simulink model "control_mixing_s"  (R2014b)
settings: Solver=ode45  SolverMode=SingleTasking  StartTime=0.0  StopTime=10.0  RelTol=1e-3
settings Model: TunableVars=quadModel  TunableVarsStorageClass=Auto  Creator=magogs00  LastModifiedBy=magogs00
settings DataIOCC: SaveFormat=Structure  SaveOutput=off  SaveTime=off
settings OptimizationCC: BlockReduction=off  BooleanDataType=off  InlineParams=on
settings DebuggingCC: UnderspecifiedInitializationDetection=Classic  MergeDetectMultiDrivingBlocksExec=none  SignalResolutionControl=TryResolveAll

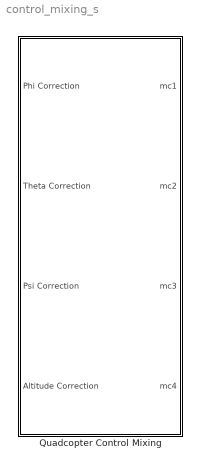
== system control_mixing_s ==
  Quadcopter Control Mixing : Subsystem
      mask help: Simulink:masks:GenSFuncDesc_MD
      mask Help: eval('feval(''rtwprivate'',''rtwhelpview'',''rtw_sfcn_block'')');
      mask Display:
      | modelLoaded = evalin('base','exist(''quadModel'',''var'')');
      | if (modelLoaded==1)
      |     if (evalin('base','quadModel.plusConfig'))
      |     fprintf([' \n' ' \n'  'Configuration "+"']);
      |     else if (~evalin('base','quadModel.plusConfig'))
      |         fprintf([' \n' ' \n' 'Configuration "X"']);
      |         end
      |     end
      | else
      |     fprintf([' \n' ' \n'  'Model Not Loaded']);
      | end

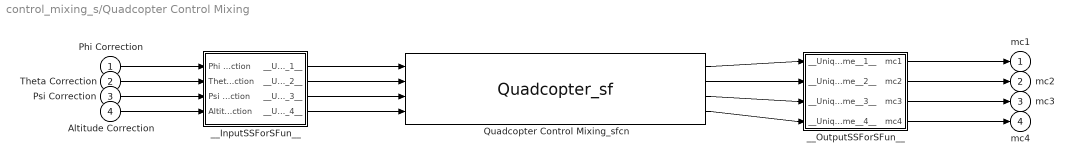
== system control_mixing_s/Quadcopter Control Mixing ==
  Phi Correction : Inport
  Theta Correction : Inport  Port=2
  Psi Correction : Inport  Port=3
  Altitude Correction : Inport  Port=4
  Quadcopter Control Mixing_sfcn : S-Function  FunctionName=Quadcopter_sf  SFunctionModules=""  EnableBusSupport=off  mask{rtw_sf_name=Quadcopter_sf, showVar=off}
      mask prompts: rtw_sf_name "Simulink:masks:GenSFuncName_MP"; showVar "Simulink:masks:GenSFuncShowModuleList_MP"
      mask help: Simulink:masks:GenSFuncDesc_MD
      mask init:
      | displist = '';
      | if ~strcmp(get_param(gcb, 'FunctionName'), rtw_sf_name);
      |   set_param(gcb, 'FunctionName', rtw_sf_name);
      | end
      | % Check if we are generating code
      | rtw_mode = false;
      | if strcmpi(get_param(bdroot(gcb),'SimulationStatus'),'Initializing')
      | 	rtw_mode = strcmpi(get_param(bdroot(gcb),'BuildingRTWCode'),'on') && ...
      | 		~strcmpi(get_param(bdroot(gcb),'TargetStyle'),'SimulationTarget');
      | end
      | if showVar || rtw_mode
      | 	if exist('rtwsfunc') == 2 | exist('rtwsfunc') == 6
      | 		tmplist = rtwsfunc(rtw_sf_name,gcb);
      | 		tmplist = DAStudio.message('Simulink:masks:GenSFuncListOfModules_IC', tmplist);
      | 	elseif showVar
      | 		tmplist1 = DAStudio.message('Simulink:masks:GenSFuncListOfModules_IC', '');
      |         tmplist2 = DAStudio.message('Simulink:masks:GenSFuncNotLicensed_IC');
      |         tmplist = [tmplist1 tmplist2];
      |  	end
      | end
      | if showVar
      |   displist = tmplist;
      | end
      settings: CopyFcn=|
      | if ~strcmp(get_param(gcb,'Linkstatus'),'none') && ...
      | ~strcmp(get_param(gcb,'Linkstatus'),'implicit')
      |   set_param(gcb,'LinkStatus','none');
      | end
      mask Help: eval('feval(''rtwprivate'',''rtwhelpview'',''rtw_sfcn_block'')');
      mask Display:
      | port_label('input',1,'Phi Correction');
      | port_label('input',2,'Theta Correction');
      | port_label('input',3,'Psi Correction');
      | port_label('input',4,'Altitude Correction');
      | port_label('output',1,'mc1');
      | port_label('output',2,'mc2');
      | port_label('output',3,'mc3');
      | port_label('output',4,'mc4');
  __InputSSForSFun__ : Subsystem
  __OutputSSForSFun__ : Subsystem
  mc1 : Outport
  mc2 : Outport  Port=2
  mc3 : Outport  Port=3
  mc4 : Outport  Port=4
  wires:
  Phi Correction/1 -> __InputSSForSFun__/1(Phi Correction)
  Theta Correction/1 -> __InputSSForSFun__/2(Theta Correction)
  Psi Correction/1 -> __InputSSForSFun__/3(Psi Correction)
  Altitude Correction/1 -> __InputSSForSFun__/4(Altitude Correction)
  __InputSSForSFun__/1(__UniqueOutportName__1__) -> Quadcopter Control Mixing_sfcn/1
  __InputSSForSFun__/2(__UniqueOutportName__2__) -> Quadcopter Control Mixing_sfcn/2
  __InputSSForSFun__/3(__UniqueOutportName__3__) -> Quadcopter Control Mixing_sfcn/3
  __InputSSForSFun__/4(__UniqueOutportName__4__) -> Quadcopter Control Mixing_sfcn/4
  Quadcopter Control Mixing_sfcn/1 -> __OutputSSForSFun__/1(__UniqueInportName__1__)
  Quadcopter Control Mixing_sfcn/2 -> __OutputSSForSFun__/2(__UniqueInportName__2__)
  Quadcopter Control Mixing_sfcn/3 -> __OutputSSForSFun__/3(__UniqueInportName__3__)
  Quadcopter Control Mixing_sfcn/4 -> __OutputSSForSFun__/4(__UniqueInportName__4__)
  __OutputSSForSFun__/1(mc1) -> mc1/1
  __OutputSSForSFun__/2(mc2) -> mc2/1
  __OutputSSForSFun__/3(mc3) -> mc3/1
  __OutputSSForSFun__/4(mc4) -> mc4/1

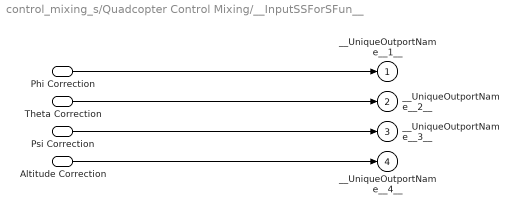
== system control_mixing_s/Quadcopter Control Mixing/__InputSSForSFun__ ==
  Phi Correction : Inport
  Theta Correction : Inport  Port=2
  Psi Correction : Inport  Port=3
  Altitude Correction : Inport  Port=4
  __UniqueOutportName__1__ : Outport
  __UniqueOutportName__2__ : Outport  Port=2
  __UniqueOutportName__3__ : Outport  Port=3
  __UniqueOutportName__4__ : Outport  Port=4
  wires:
  Phi Correction/1 -> __UniqueOutportName__1__/1
  Theta Correction/1 -> __UniqueOutportName__2__/1
  Psi Correction/1 -> __UniqueOutportName__3__/1
  Altitude Correction/1 -> __UniqueOutportName__4__/1

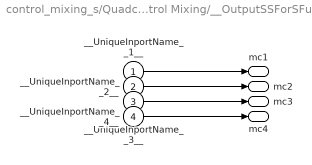
== system control_mixing_s/Quadcopter Control Mixing/__OutputSSForSFun__ ==
  __UniqueInportName__1__ : Inport
  __UniqueInportName__2__ : Inport  Port=2
  __UniqueInportName__3__ : Inport  Port=3
  __UniqueInportName__4__ : Inport  Port=4
  mc1 : Outport
  mc2 : Outport  Port=2
  mc3 : Outport  Port=3
  mc4 : Outport  Port=4
  wires:
  __UniqueInportName__1__/1 -> mc1/1
  __UniqueInportName__2__/1 -> mc2/1
  __UniqueInportName__3__/1 -> mc3/1
  __UniqueInportName__4__/1 -> mc4/1
